simulink model "session2"  (R2024b)
settings: Solver=FixedStepAuto  StartTime=0.0  StopTime=10.0  FixedStep=0.001  RelTol=1e-3
values from neighbouring files (symbols this model uses):
  Cd = [0 1]    [mpc3.m]
  Cr = 87342    [mpc3.m]    (also in prueba_mpc.m; prueba_mpc2.m)
  m = 1400    [mpc3.m]    (also in prueba_mpc.m; prueba_mpc2.m)
  R = 1    [prueba_mpc.m]    (also in prueba_mpc2.m)
  vx = 10    [mpc3.m]    (also in prueba_mpc.m; prueba_mpc2.m)
undefined symbols (not defined in the file or in its folder): Af, C_lambda, F_max, FN, g, mode, mu1, mu2, mu3, omega, theta
libraries: slpidlib x1
settings Model: Creator=inaki  LastModifiedBy=inaki
settings DebuggingCC: AlgebraicLoopMsg=none

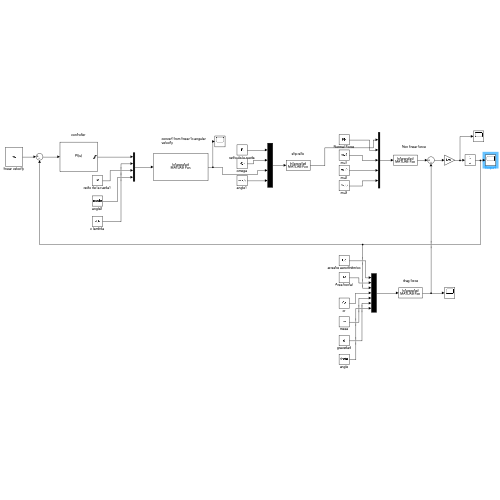
[thumbnail: Simulink's stored preview of the top-level diagram]
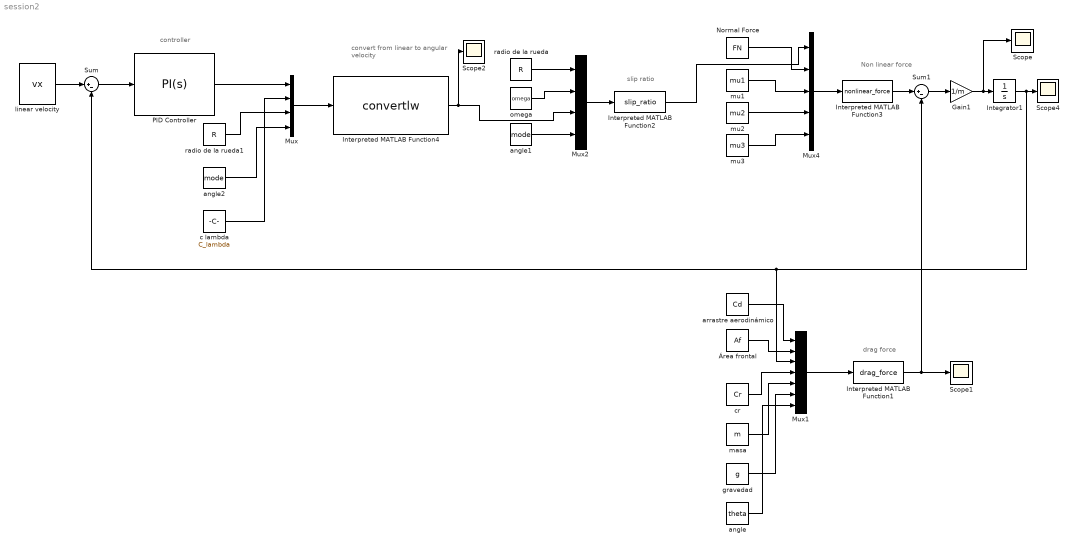
== system session2 ==
  note: controller
  note: Non linear force
  note: slip ratio
  note: drag force
  note: convert from linear to angular velocity
  Gain1 : Gain  Gain=1/m
  Integrator1 : Integrator  UpperSaturationLimit=50  LowerSaturationLimit=0
  Interpreted MATLAB Function1 : MATLABFcn  MATLABFcn=drag_force  OutputDimensions=1  Output1D=off
  Interpreted MATLAB Function2 : MATLABFcn  MATLABFcn=slip_ratio  Output1D=off
  Interpreted MATLAB Function3 : MATLABFcn  MATLABFcn=nonlinear_force  OutputDimensions=1  Output1D=off
  Interpreted MATLAB Function4 : MATLABFcn  MATLABFcn=convertlw  Output1D=off
  Mux : Mux
  Mux1 : Mux  Inputs=7
  Mux2 : Mux
  Mux4 : Mux  Inputs=5
  Normal Force : Constant  Value=FN
  PID Controller : slpidlib/PID Controller  Controller=PI  Form=Parallel  TimeDomain=Continuous-time  UseExternalTs=off  SampleTime=-1  IntegratorMethod=Forward Euler  FilterMethod=Forward Euler  ControllerParametersSource=internal  P=0.1  I=0.05  UseKiTs=off  D=0  UseExternalDerivativeSource=off  N=100  UseFilter=on  TunerSelectOption=Transfer Function Based (PID Tuner App)  InitialConditionSource=internal  InitialConditionForIntegrator=0  InitialConditionForFilter=0  DifferentiatorICPrevScaledInput=0  ExternalReset=none  TrackingMode=off  Kt=1  LimitOutput=on  SatLimitsSource=internal  UpperSaturationLimit=F_max  LowerSaturationLimit=-F_max  LinearizeAsGain=on  AntiWindupMode=clamping  Kb=1  LimitIntegrator=on  UpperIntegratorSaturationLimit=50  LowerIntegratorSaturationLimit=0  POutMin=[]  POutMax=[]  IOutMin=[]  IOutMax=[]  DOutMin=[]  DOutMax=[]  NOutMin=[]  NOutMax=[]  SumOutMin=[]  SumOutMax=[]  SaturationOutMin=[]  SaturationOutMax=[]  PParamMin=[]  PParamMax=[]  IParamMin=[]  IParamMax=[]  DParamMin=[]  DParamMax=[]  NParamMin=[]  NParamMax=[]  KbParamMin=[]  KbParamMax=[]  KtParamMin=[]  KtParamMax=[]  KbOutMin=[]  KbOutMax=[]  KtOutMin=[]  KtOutMax=[]  IntegratorOutMin=[]  IntegratorOutMax=[]  FilterOutMin=[]  FilterOutMax=[]  SumI1OutMin=[]  SumI1OutMax=[]  SumI2OutMin=[]  SumI2OutMax=[]  SumI3OutMin=[]  SumI3OutMax=[]  SumI4OutMin=[]  SumI4OutMax=[]  SumDOutMin=[]  SumDOutMax=[]  DifferentiatorOutMin=[]  DifferentiatorOutMax=[]  FilterDiffOutCoefMin=[]  FilterDiffOutCoefMax=[]  ReciprocalOutMin=[]  ReciprocalOutMax=[]  SumDenOutMin=[]  SumDenOutMax=[]  SumNumOutMin=[]  SumNumOutMax=[]  DivideOutMin=[]  DivideOutMax=[]  UdiffTsProdOutMin=[]  UdiffTsProdOutMax=[]  NTsProdOutMin=[]  NTsProdOutMax=[]  UintegralTsProdOutMin=[]  UintegralTsProdOutMax=[]  UngainTsProdOutMin=[]  UngainTsProdOutMax=[]  ClampingZeroOutDataTypeStr=Inherit: Inherit via back propagation  ClampingZeroOutMin=[]  ClampingZeroOutMax=[]  FilterDenConstantOutDataTypeStr=Inherit: Inherit via back propagation  FilterDenConstantOutMin=[]  FilterDenConstantOutMax=[]  PCopyOutDataTypeStr=Inherit: Inherit via back propagation  PCopyOutMin=[]  PCopyOutMax=[]  NCopyOutDataTypeStr=Inherit: Inherit via back propagation  NCopyOutMin=[]  NCopyOutMax=[]  IntegratorContinuousStateAttributes=''  IntegratorStateMustResolveToSignalObject=off  IntegratorRTWStateStorageClass=Auto  FilterContinuousStateAttributes=''  FilterStateMustResolveToSignalObject=off  FilterRTWStateStorageClass=Auto  ParallelPVariant=InternalParameters  IdealPVariant=Disabled  IVariant=InternalParameters  DVariant=Disabled  IntegratorVariant=Continuous  SatVariant=Enabled  AWVariant=ContClampingParallel  PCopyVariant=Disabled  TRVariant=Disabled  FdbkBlocksVariant=Forward  IdealPFdbkVariant=Disabled  SatFdbkVariant=Disabled  DerivativeFilterVariant=Disabled  NVariant=Disabled  NCopyVariant=Disabled_SignalSpec  FilterICVariant=Disabled  IntegratorICVariant=InternalICs  ExternalResetVariant=Disabled  TRSumVariant=Passthrough  SumFdbkVariant=Disabled  SumVariant=Sum_PI  TsampFilterVariant=InternalTs  TsampNgainVariant=Passthrough  TsampIntegralVariant=Disabled_SignalSpec  ExternalSaturationOutDataTypeStr=Inherit: Same as second input  DerivativeSourceVariant=Disabled  PreIntVariant=InternalPreInt
  Scope{,1..2,4} (4 alike) : Scope
  Sum : Sum  Inputs=|+-
  Sum1 : Sum  Inputs=|+-
  angle : Constant  Value=theta  VectorParams1D=off
  angle1 : Constant  Value=mode
  angle2 : Constant  Value=mode
  arrastre aerodinámico : Constant  Value=Cd  VectorParams1D=off
  c lambda : Constant  Value=C_lambda
  cr : Constant  Value=Cr  VectorParams1D=off
  gravedad : Constant  Value=g  VectorParams1D=off
  linear velocity : Constant  Value=vx  SampleTime=vx
  masa : Constant  Value=m  VectorParams1D=off
  mu1 : Constant  Value=mu1
  mu2 : Constant  Value=mu2
  mu3 : Constant  Value=mu3
  omega : Constant  Value=omega  VectorParams1D=off
  radio de la rueda : Constant  Value=R  VectorParams1D=off
  radio de la rueda1 : Constant  Value=R  VectorParams1D=off
  Área frontal : Constant  Value=Af  VectorParams1D=off
  wires:
  Mux1/1 -> Interpreted MATLAB Function1/1
  Área frontal/1 -> Mux1/2
  gravedad/1 -> Mux1/6
  arrastre aerodinámico/1 -> Mux1/1
  angle1/1 -> Mux2/4
  mu2/1 -> Mux4/4
  cr/1 -> Mux1/4
  masa/1 -> Mux1/5
  Mux4/1 -> Interpreted MATLAB Function3/1
  Mux2/1 -> Interpreted MATLAB Function2/1
  Sum1/1 -> Gain1/1
  angle/1 -> Mux1/7
  Gain1/1 -> Scope/1, Integrator1/1
  omega/1 -> Mux2/2
  Interpreted MATLAB Function1/1 -> Sum1/2, Scope1/1
  mu1/1 -> Mux4/3
  mu3/1 -> Mux4/5
  radio de la rueda/1 -> Mux2/1
  Interpreted MATLAB Function2/1 -> Mux4/1
  Normal Force/1 -> Mux4/2
  linear velocity/1 -> Sum/1
  Interpreted MATLAB Function4/1 -> Scope2/1, Mux2/3
  Mux/1 -> Interpreted MATLAB Function4/1
  radio de la rueda1/1 -> Mux/3
  angle2/1 -> Mux/4
  c lambda/1 -> Mux/2
  PID Controller/1 -> Mux/1
  Integrator1/1 -> Scope4/1, Sum/2, Mux1/3
  Interpreted MATLAB Function3/1 -> Sum1/1
  Sum/1 -> PID Controller/1
